simulink model "V126_L8_UMS"  (R2020b)
settings: Solver=VariableStepAuto  StartTime=0.0  StopTime=100  MaxStep=0.04  RelTol=1e-3
undefined symbols (not defined in the file): Ad, Bd, Cd, Dd, F, K, K1, K2, Kg, L, m0, m1, m2, n0, n1, n2, q, T1, T2, T3, Ts, Un
settings Model: Creator=td  LastModifiedBy=Maxim
settings DataIOCC: ReturnWorkspaceOutputs=off
settings DebuggingCC: ArithmeticOperatorsInVariantConditions=warning
settings SFSimCC: CustomCodeUndefinedFunction=UseInterfaceOnly

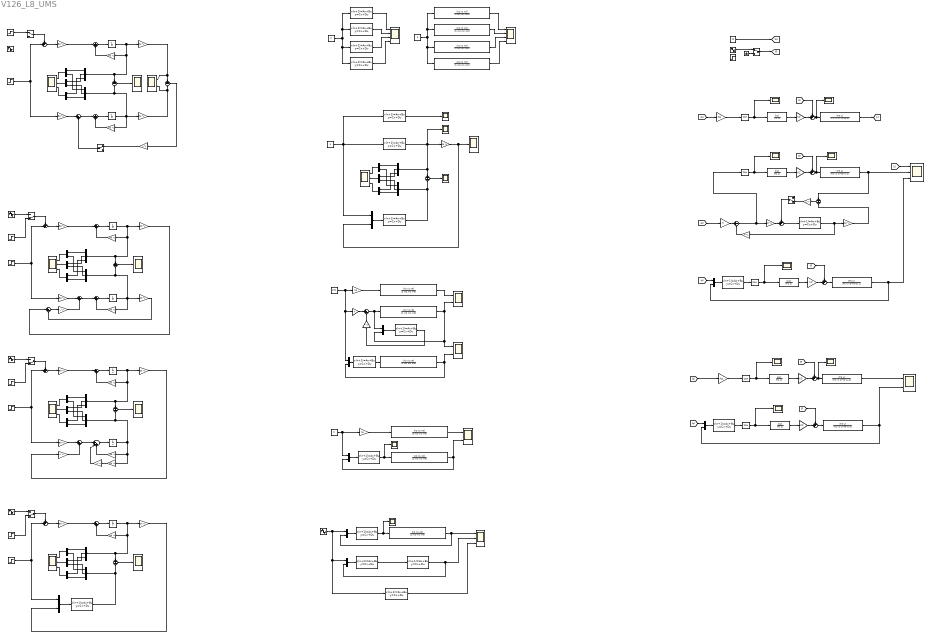
== system V126_L8_UMS ==
  note: Помилка   спостереження
      | вектору     стану
  note: Реальний та спостережений стан об’єкта:
  note: u[n]
  note: ey[n]
  note: x[n+1] = Ad*x[n] + Bd*(u[n]+f[n])
      | y[n] = Cd*x[n]
  note: Збурення f[n]
  note: Модель об'єкта в Просторі Станів
  note: u(t)
  note: V=126; T1=4; T2=6; q=0.3; T3=0.8; K1=0.3; K2=0.2; Un=100;
      |
      | Pn = 6 Bar
      | Rn = 30 rps
      |
      | g = 0.5*Pn = 15 Bar
  note: Вхідні сигнали:
      |
      | g - уставка тиску
      |
      | f - збурення
  note: Об'єкт керування (plant)
  note: Об'єкт керування (plant)
  note: u(t)
  note: xo[n]
  note: Цифрова модель Об'єкта керування (plant) в Просторі Станів
  note: u[n]
  note: Модальний регулятор
  note: u[n]
  note: xo[n+1]
  note: xo[n]
  note: x[n+1]
  note: x[n]
  note: Сигнал
      | керування
  note: y[n]
  note: yo[n]
  note: Спостерігач стану: [Цифровий двійник] + [Корекція помилки спостереження]
  note: ey[n]
  note: ex[n]
  note: x[n]
  note: x[n+1]
  note: xo[n]
  note: xo[n+1]
  note: Модель об'єкта в Просторі Станів
  note: ex[n]
  note: y[n]
  note: Спостерігач стану: [Цифровий двійник] + [Корекція помилки спостереження]
  note: ey[n]
  note: Збурення f[n]
  note: yo[n]
  note: Сигнал
      | керування
  note: x[n+1] = Ad*x[n] + Bd*(u[n]+f[n])
      | y[n] = Cd*x[n]
  note: u[n]
  note: ex[n] = x[n] - xo[n]
      |
      | x[n+1] = A*x[n] + B*u[n]
      | xo[n+1] = A*xo[n] + B*u[n] + L*C*x[n] - L*C*xo[n]
      |
      | x[n+1] - xo[n+1] = A*x[n] + B*u[n] - A*xo[n] - B*u[n] - L*C*x[n] + L*C*xo[n]
      |
      | x[n+1] - xo[n+1] = A*x[n] - L*C*x[n] - A*xo[n] + L*C*xo[n]
      |
      | x[n+1] - xo[n+1] = A*x[n] - L*C*x[n] - (A*xo[n] - L*C*xo[n])
      |
      | x[n+1] - xo[n+1] = (A - L*C)* (x[n] - xo[n])
      |
      | ex[n+1] = (A - L*C)* ex[n]
  note: x[n+1] = A*x[n] + B*u[n]
      | y[n] = C*x[n]
      |
      | xo[n+1] = A*xo[n] + B*u[n]
      | yo[n] = C*xo[n]
  note: xo[n+1] = A*xo[n] + B*u[n] + L (y[n] - yo[n])
      | yo[n] = C*xo[n]
      |
      | xo[n+1] = A*xo[n] + B*u[n] + L (C*x[n] - C*xo[n])
      |
      | xo[n+1] = A*xo[n] + B*u[n] + L*C*x[n] - L*C*xo[n]
      |
      | xo[n+1] = (A - L*C)*xo[n] + B*u[n] + L*C*x[n]
  note: ex[n]
  note: Модель об'єкта в Просторі Станів
  note: xo[n+1]
  note: Спостерігач стану: [Цифровий двійник] + [Корекція помилки спостереження]
  note: y[n]
  note: x[n+1]
  note: x[n]
  note: Сигнал
      | керування
  note: Збурення f[n]
  note: u[n]
  note: xo[n]
  note: x[n+1] = Ad*x[n] + Bd*(u[n]+f[n])
      | y[n] = Cd*x[n]
  note: y[n]
  note: xo[n]
  note: x[n]
  note: xo[n]
  note: Сигнал
      | керування
  note: Спостерігач стану.
  note: y[n]
  note: Збурення f[n]
  note: Модель об'єкта в Просторі Станів
  note: ex[n]
  note: x[n+1] = Ad*x[n] + Bd*(u[n]+f[n])
      | y[n] = Cd*x[n]
  note: y[n]
  note: u[n]
  note: x[n]
  note: x[n]
  note: x[n+1]
  note: xo[n]
  note: ex[n]
  note: x[n]
  note: xo[n]
  note: xo[n]
  note: Спостерігач стану.
  note: x[n]
  note: xo[n]
  note: xo[n+1] = (A - L*C)*xo[n] + B*u[n] + L*y[n]
      | yo[n] = xo[n]
      |
      | ---------------------------------------------------------
      | yr[n] = u[n] = K*g[n] - F*xo[n]
      |
      | xo[n+1] = (A - L*C)*xo[n] + B*(K*g[n] - F*xo[n]) + L*y[n]
      | xo[n+1] = (A - L*C)*xo[n] + B*K*g[n] - B*F*xo[n] + L*y[n]
      |
      | xo[n+1] = (A - L*C-B*F)*xo[n] + B*K*g[n] + L*y[n]
      | yr[n] = -F*xo[n] + K*g[n] + 0*y[n]
  note: u[n]
  note: y[n]
  note: g[n]
  note: u[n]
  note: Об'єкт керування (plant)
  note: u(t)
  note: u[n]
  note: g[n]
  note: y[n]
  note: x[n+1] = Ad*x[n] + Bd*yr[n]
      | y[n] = Cd*x[n]
      |
      | xo[n+1] = (Ad - L*Cd - Bd*F)*xo[n] + Bd*K*u[n] + L*y[n]
      | yr[n] = -F*xo[n] + K*u[n]
      |
      | -------------------------------------------------------------------------------------
      |
      | x[n+1] = Ad*x[n] - Bd*F*xo[n] + Bd*K*u[n]
      | xo[n+1] = L*Cd*x[n] (Ad - L*Cd - Bd*F)*xo[n] + Bd*K*u[n]
      |
      | y[n] = Cd*x[n] + [0,0,0] *xo[n]
  note: u[n]
  note: y[n]
  note: u[n]
  note: y[n]
  note: y[n]
  note: yr[n]
  note: u(t)
  note: Об'єкт керування (plant)
  note: Об'єкт керування (plant)
  note: u(t)
  "    Wpump (s) " : TransferFcn  Numerator=[T3 1]  Denominator=[T2^2 (2*T2*q) 1]
  "    Wpump (s)  " : TransferFcn  Numerator=[T3 1]  Denominator=[T2^2 (2*T2*q) 1]
  "  Wengine (s)  " : TransferFcn  Numerator=[K1]  Denominator=[T1 1]
  "  Wengine (s)   " : TransferFcn  Numerator=[K1]  Denominator=[T1 1]
  "  Wpump (s)" : TransferFcn  Numerator=[T3 1]  Denominator=[T2^2 (2*T2*q) 1]
  "  Wpump (s) " : TransferFcn  Numerator=[T3 1]  Denominator=[T2^2 (2*T2*q) 1]
  "  Wpump (s)   " : TransferFcn  Numerator=[T3 1]  Denominator=[T2^2 (2*T2*q) 1]
  "  y[n]  " : Scope  NumInputPorts=2
  " Plant Model State Space" : DiscreteStateSpace  A=Ad  B=Bd  C=eye(3)  D=[0;0;0]  InitialCondition=[-682.44; 264.94; 115.78]  SampleTime=Ts
  " Plant Model State Space " : DiscreteStateSpace  A=Ad  B=Bd  C=Cd  D=Dd  InitialCondition=[-682.44; 264.94; 115.78]  SampleTime=Ts
  " Plant Model TF " : DiscreteTransferFcn  Numerator=[n2 n1 n0]  Denominator=[1 m2 m1 m0]  InitialStates=[115.78; 264.94; -682.44]  SampleTime=Ts
  " Plant Model TF   " : DiscreteTransferFcn  Numerator=[n2 n1 n0]  Denominator=[1 m2 m1 m0]  InitialStates=[115.78; 264.94; -682.44]  SampleTime=Ts
  " Plant Model TF   1" : DiscreteTransferFcn  Numerator=[n2 n1 n0]  Denominator=[1 m2 m1 m0]  InitialStates=[115.78, 264.94, -682.44]  SampleTime=Ts
  " Plant Model TF   2" : DiscreteTransferFcn  Numerator=[n2 n1 n0]  Denominator=[1 m2 m1 m0]  InitialStates=[0, 0, -1456.6]  SampleTime=Ts
  " Plant Model TF   3" : DiscreteTransferFcn  Numerator=[n2 n1 n0]  Denominator=[1 m2 m1 m0]  InitialStates=[0, 763.7678, 0]  SampleTime=Ts
  " Plant Model TF   4" : DiscreteTransferFcn  Numerator=[n2 n1 n0]  Denominator=[1 m2 m1 m0]  InitialStates=[ 627.2564, 0, 0]  SampleTime=Ts
  " Plant Model1" : DiscreteStateSpace  A=Ad  B=Bd  C=Cd  D=Dd  InitialCondition=[-682.44; 264.94; 115.78]  SampleTime=Ts
  " Plant Model2" : DiscreteStateSpace  A=Ad  B=Bd  C=Cd  D=Dd  InitialCondition=[-1456.6; 0; 0]  SampleTime=Ts
  " Plant Model3" : DiscreteStateSpace  A=Ad  B=Bd  C=Cd  D=Dd  InitialCondition=[0; 763.7678; 0]  SampleTime=Ts
  " Plant Model4" : DiscreteStateSpace  A=Ad  B=Bd  C=Cd  D=Dd  InitialCondition=[0; 0; 627.2564]  SampleTime=Ts
  " R = Observer + ModReg" : DiscreteStateSpace  A=Ad - L*Cd - Bd*F  B=[Bd*K, L]  C=-F  D=[K, 0 ]  SampleTime=Ts
  " System" : DiscreteStateSpace  A=[ Ad, -Bd*F; L*Cd, (Ad - L*Cd - Bd*F)]  B=[Bd*K; Bd*K]  C=[Cd, 0, 0, 0]  D=[0]  InitialCondition=[-682.44; 264.94; 115.78; 0; 0; 0]  SampleTime=Ts
  " u[n] " : Scope
  " y[n]" : Scope
  " y[n]1" : Scope  NumInputPorts=4
  " y[n]2" : Scope  NumInputPorts=2
  " y[n]3" : Scope  NumInputPorts=2
  " y[n]6" : Scope  NumInputPorts=3
  " y[n]7" : Scope
  " y[n]8" : Scope  NumInputPorts=4
  " Порівняльник  " : Scope  NumInputPorts=2
   Порівняльник {1,3,5,8..9,11,13..21} (15 alike) : Scope
   Порівняльник {2,6..7,10,12} (5 alike) : Scope  NumInputPorts=3
  " Порівняльник 4" : Scope  NumInputPorts=2
  -C1 : Step  Time=26  After=-4  SampleTime=0
  -K*Un : Step  Time=26  After=-0.4*Un  SampleTime=0
  Cl/Op Loop Obs : ManualSwitch
  Constant : Constant  Value=0
  Constant1 : Constant  Value=0
  Constant2 : Constant  Value=0
  Constant3 : Constant  Value=12
  Demux{2..11} (10 alike) : Demux  Outputs=3
  Gain{,5,7,9,39} (5 alike) : Gain  Gain=K2
  Gain{1,4,6,8} (4 alike) : Gain  Gain=Kg
  Gain{2,10,12,17,22,24,29,31,37} (9 alike) : Gain  Gain=Cd  Multiplication=Matrix(K*u)
  Gain{11,16,19,23,26,30,33,40} (8 alike) : Gain  Gain=Bd  Multiplication=Matrix(K*u)
  Gain{13,18,25,32,36} (5 alike) : Gain  Gain=L  Multiplication=Matrix(K*u)
  Gain14 : Gain  Gain=F  Multiplication=Matrix(K*u)
  Gain15 : Gain  Gain=K
  Gain{20..21,27..28,34..35,41} (7 alike) : Gain  Gain=Ad  Multiplication=Matrix(K*u)
  Gain3 : Gain  Gain=F  Multiplication=Matrix(K*u)
  Gain38 : Gain  Gain=K
  Ground : Ground
  Manual Switch1 : ManualSwitch
  Manual Switch2 : ManualSwitch
  Manual Switch{3..6} (4 alike) : ManualSwitch  CurrentSetting=0
  Mux{,1..23} (24 alike) : Mux  Inputs=2
  Observer : DiscreteStateSpace  A=Ad-L*Cd  B=[Bd, L]  C=eye(3)  D=[0 0; 0 0; 0 0 ]  SampleTime=Ts
  "Observer " : DiscreteStateSpace  A=Ad-L*Cd  B=[Bd, L]  C=eye(3)  D=[0 0; 0 0; 0 0 ]  SampleTime=Ts
  Observer Cl_Loop : DiscreteStateSpace  A=Ad-L*Cd  B=[Bd, L]  C=eye(3)  D=[0 0; 0 0; 0 0 ]  SampleTime=Ts
  Observer Op_Loop : DiscreteStateSpace  A=Ad  B=Bd  C=eye(3)  D=[0;0;0]  SampleTime=Ts
  Plant Model TF : DiscreteTransferFcn  Numerator=[n2 n1 n0]  Denominator=[1 m2 m1 m0]  InitialStates=[115.78; 264.94; -682.44]  SampleTime=Ts
  "Plant Model TF " : DiscreteTransferFcn  Numerator=[n2 n1 n0]  Denominator=[1 m2 m1 m0]  InitialStates=[115.78; 264.94; -682.44]  SampleTime=Ts
  "Plant Model TF    " : DiscreteTransferFcn  Numerator=[n2 n1 n0]  Denominator=[1 m2 m1 m0]  InitialStates=[115.78; 264.94; -682.44]  SampleTime=Ts
  "Plant Model TF     " : DiscreteTransferFcn  Numerator=[n2 n1 n0]  Denominator=[1 m2 m1 m0]  InitialStates=[115.78; 264.94; -682.44]  SampleTime=Ts
  R = Observer + ModReg : DiscreteStateSpace  A=Ad - L*Cd - Bd*F  B=[Bd*K, L]  C=-F  D=[K, 0 ]  SampleTime=Ts
  "R = Observer + ModReg " : DiscreteStateSpace  A=Ad - L*Cd - Bd*F  B=[Bd*K, L]  C=-F  D=[K, 0 ]  SampleTime=Ts
  "R = Observer + ModReg  " : DiscreteStateSpace  A=Ad - L*Cd - Bd*F  B=[Bd*K, L]  C=-F  D=[K, 0 ]  SampleTime=Ts
  R = Observer + ModReg1 : DiscreteStateSpace  A=Ad - L*Cd - Bd*F  B=[Bd*K, L]  C=-F  D=[K, 0 ]  SampleTime=Ts
  R = Observer + ModReg2 : DiscreteStateSpace  A=Ad - L*Cd - Bd*F  B=[Bd*K, L]  C=-F  D=[K, 0 ]  SampleTime=Ts
  Sine Wave : Sin  Amplitude=2  Frequency=0.4  SampleTime=Ts
  Sine Wave{2..5} (4 alike) : Sin  Amplitude=8  Frequency=0.2  SampleTime=Ts
  Sine Wave6 : Sin  Amplitude=4  Frequency=0.2  SampleTime=0
  Sum : Sum  Inputs=|+-
  Sum{1..2,4..5,7,9..10,21,27,31} (10 alike) : Sum  Inputs=++|
  Sum{11..12,14,16..17,19,22,25,29} (9 alike) : Sum  Inputs=|++
  Sum{3,6,13,15,20,26,30} (7 alike) : Sum  Inputs=+|-
  Sum18 : Sum  Inputs=|+-
  Sum23 : Sum  Inputs=||+-+
  Sum8 : Sum  Inputs=|+-
  Un{,1..2,4} (4 alike) : Step  Time=0  After=Un  SampleTime=0
  Un3 : Step  Time=26  After=-0.4*Un  SampleTime=0
  Un5 : Step  Time=26  After=-0.4*Un  SampleTime=0
  Un6 : Step  Time=26  After=-0.4*Un  SampleTime=0
  Unit Delay{1..6,8} (7 alike) : UnitDelay  SampleTime=Ts  HasFrameUpgradeWarning=on
  "Wengine (s) " : TransferFcn  Numerator=[K1]  Denominator=[T1 1]
  "Wengine (s)  " : TransferFcn  Numerator=[K1]  Denominator=[T1 1]
  "Wengine (s)   " : TransferFcn  Numerator=[K1]  Denominator=[T1 1]
  ZOH : ZeroOrderHold  SampleTime=Ts
  ZOH :) : ZeroOrderHold  SampleTime=Ts
  ZOH :)1 : ZeroOrderHold  SampleTime=Ts
  "ZOH " : ZeroOrderHold  SampleTime=Ts
  ZOH1 : ZeroOrderHold  SampleTime=Ts
  g : Constant  Value=100
  g1 : Constant  Value=0
  x[n+1]=Ad*x[n+1] : DiscreteStateSpace  A="[ 0 1 0 ; 0 0 1 ;  -m0  -m1  -m2 ]"  B=[1 0 0; 0 1 0; 0 0 1]  C=[1 0 0; 0 1 0; 0 0 1]  D=[0 0 0; 0 0 0; 0 0 0]  SampleTime=Ts
  Порівняльник1 : Scope  NumInputPorts=3
  wires:
  Sine Wave6/1 -> Manual Switch1/1
  Gain/1 -> Sum10/2
  Sum10/1 -> " Порівняльник 18"/1, "  Wpump (s)"/1
  Manual Switch1/1 -> [f]
  "  Wpump (s)"/1 -> [y]
  [f] -> Sum10/1
  Constant3/1 -> [g]
  "Wengine (s) "/1 -> Gain/1
  ZOH/1 -> "Wengine (s) "/1, " Порівняльник 3"/1
  Ground/1 -> Manual Switch1/2
  [g] -> Gain1/1
  Gain1/1 -> ZOH/1
  Manual Switch6/1 -> Sum7/1
  "    Wpump (s) "/1 -> Порівняльник1/3, Mux20/2
  Gain9/1 -> Sum5/2
  "Wengine (s)   "/1 -> Gain9/1
  "  Wpump (s)   "/1 -> Порівняльник1/2, Sum6/1
  Gain12/1 -> Sum6/2
  Sum5/1 -> " Порівняльник 17"/1, "  Wpump (s)   "/1
  Gain11/1 -> Sum7/2
  x[n+1]=Ad*x[n+1]/1 -> Gain14/1, Gain12/1
  Sum6/1 -> Gain13/1
  [f] -> Sum5/1
  "ZOH "/1 -> "Wengine (s)   "/1, " Порівняльник 1"/1
  Sum7/1 -> x[n+1]=Ad*x[n+1]/1
  Sum8/1 -> Gain11/1, "ZOH "/1
  Gain14/1 -> Sum8/2
  [g] -> Gain15/1
  Gain15/1 -> Sum8/1
  Unit Delay2/1 -> Gain20/1, Demux2/1, Sum15/1, Gain10/1
  Gain10/1 -> " Порівняльник 4"/1, Sum13/1
  Un/1 -> Sum9/2, Gain16/1
  Unit Delay1/1 -> Demux3/1, Sum15/2, Gain17/1, Gain21/1
  Gain17/1 -> " Порівняльник 4"/2, Sum13/2
  Gain21/1 -> Sum12/2
  Sum11/1 -> Sum12/1
  Sum12/1 -> Unit Delay1/1
  Gain16/1 -> Sum11/1
  -K*Un/1 -> Manual Switch2/1
  Sum9/1 -> Gain19/1
  Manual Switch2/1 -> Sum9/1
  Demux2/1 -> Mux/1
  Demux3/1 -> Mux/2
  Mux/1 -> " Порівняльник 2"/1
  Mux1/1 -> " Порівняльник 2"/2
  Demux3/3 -> Mux2/2
  Mux2/1 -> " Порівняльник 2"/3
  Demux2/3 -> Mux2/1
  Demux2/2 -> Mux1/1
  Demux3/2 -> Mux1/2
  Gain18/1 -> Cl/Op Loop Obs/1
  Cl/Op Loop Obs/1 -> Sum11/2
  Sum13/1 -> Gain18/1
  Sum14/1 -> Unit Delay2/1
  Gain20/1 -> Sum14/2
  Gain19/1 -> Sum14/1
  Sum15/1 -> " Порівняльник 5"/1
  Gain23/1 -> Sum16/1
  Unit Delay4/1 -> Gain27/1, Demux4/1, Sum20/1, Gain22/1
  Gain27/1 -> Sum19/2
  Sum17/1 -> Unit Delay3/1
  Unit Delay3/1 -> Demux5/1, Sum20/2, Gain24/1, Gain28/1
  Gain28/1 -> Sum17/2
  Gain22/1 -> Sum18/1
  Un3/1 -> Manual Switch3/2
  Un2/1 -> Sum21/2, Gain23/1
  Gain26/1 -> Sum19/1
  Demux5/3 -> Mux5/2
  Mux5/1 -> " Порівняльник 6"/3
  Mux4/1 -> " Порівняльник 6"/2
  Sum20/1 -> " Порівняльник 8"/1
  Sum21/1 -> Gain26/1
  Mux3/1 -> " Порівняльник 6"/1
  Demux4/3 -> Mux5/1
  Sine Wave3/1 -> Manual Switch3/1
  Demux5/1 -> Mux3/2
  Demux4/1 -> Mux3/1
  Demux5/2 -> Mux4/2
  Demux4/2 -> Mux4/1
  Sum19/1 -> Unit Delay4/1
  Sum16/1 -> Sum17/1
  Manual Switch3/1 -> Sum21/1
  Gain25/1 -> Sum16/2
  Sum18/1 -> Gain25/1
  Gain24/1 -> Sum18/2
  Mux8/1 -> " Порівняльник 7"/3
  Gain32/1 -> Sum22/2
  Mux7/1 -> " Порівняльник 7"/2
  Gain29/1 -> Gain32/1
  Unit Delay6/1 -> Gain34/1, Demux6/1, Sum26/1, Gain29/1
  Gain34/1 -> Sum25/2
  Demux7/3 -> Mux8/2
  Unit Delay5/1 -> Demux7/1, Sum26/2, Gain37/1, Gain35/1
  Sum26/1 -> " Порівняльник 9"/1
  Gain33/1 -> Sum25/1
  Un4/1 -> Sum27/2, Gain30/1
  Manual Switch4/1 -> Sum27/1
  Sum25/1 -> Unit Delay6/1
  Sum27/1 -> Gain33/1
  Gain30/1 -> Sum22/1
  Demux6/2 -> Mux7/1
  Demux7/2 -> Mux7/2
  Sum23/1 -> Unit Delay5/1
  Demux6/1 -> Mux6/1
  Sine Wave4/1 -> Manual Switch4/1
  Demux6/3 -> Mux8/1
  Demux7/1 -> Mux6/2
  Mux6/1 -> " Порівняльник 7"/1
  Un5/1 -> Manual Switch4/2
  Sum22/1 -> Sum23/1
  Gain35/1 -> Sum23/3
  Gain37/1 -> Gain36/1
  Gain36/1 -> Sum23/2
  Unit Delay8/1 -> Gain41/1, Demux8/1, Sum30/1, Gain31/1
  Demux9/2 -> Mux10/2
  Demux8/2 -> Mux10/1
  Un6/1 -> Manual Switch5/2
  Demux8/1 -> Mux9/1
  Demux8/3 -> Mux11/1
  Manual Switch5/1 -> Sum31/1
  Sum30/1 -> " Порівняльник 11"/1
  Demux9/3 -> Mux11/2
  Demux9/1 -> Mux9/2
  Mux9/1 -> " Порівняльник 10"/1
  Gain31/1 -> Mux12/2
  Un1/1 -> Mux12/1, Sum31/2
  Mux11/1 -> " Порівняльник 10"/3
  Sum29/1 -> Unit Delay8/1
  Gain41/1 -> Sum29/2
  Mux10/1 -> " Порівняльник 10"/2
  Sine Wave2/1 -> Manual Switch5/1
  Sum31/1 -> Gain40/1
  Gain40/1 -> Sum29/1
  Mux12/1 -> Observer/1
  Observer/1 -> Sum30/2, Demux9/1
  Mux13/1 -> " Порівняльник 12"/2
  Mux14/1 -> " Порівняльник 12"/3
  Demux11/1 -> Mux16/2
  Mux16/1 -> " Порівняльник 12"/1
  Demux11/3 -> Mux14/2
  Sum3/1 -> " Порівняльник 13"/1
  Demux10/3 -> Mux14/1
  Demux10/2 -> Mux13/1
  Demux10/1 -> Mux16/1
  " Plant Model State Space"/1 -> " Порівняльник 14"/1, Demux10/1, Sum3/1, Gain2/1
  Demux11/2 -> Mux13/2
  Mux15/1 -> Observer Cl_Loop/1
  Constant/1 -> Observer Op_Loop/1, Mux15/1, " Plant Model State Space"/1
  Observer Cl_Loop/1 -> Sum3/2, Demux11/1
  Gain2/1 -> " y[n]"/1, Mux15/2
  Observer Op_Loop/1 -> " Порівняльник 15"/1
  Constant1/1 -> " Plant Model2"/1, " Plant Model1"/1, " Plant Model4"/1, " Plant Model3"/1
  " Plant Model1"/1 -> " y[n]1"/1
  " Plant Model2"/1 -> " y[n]1"/2
  " Plant Model3"/1 -> " y[n]1"/3
  " Plant Model4"/1 -> " y[n]1"/4
  g/1 -> Mux18/1, Gain38/1, Gain8/1
  Mux17/1 -> "Observer "/1
  Sum/1 -> Mux17/1, " Plant Model TF "/1
  " Plant Model TF "/1 -> " y[n]3"/1, Mux17/2, " y[n]2"/2
  Plant Model TF/1 -> " y[n]2"/1
  Gain3/1 -> Sum/2
  "Observer "/1 -> Gain3/1
  Gain8/1 -> Plant Model TF/1
  Gain38/1 -> Sum/1
  Mux18/1 -> R = Observer + ModReg/1
  R = Observer + ModReg/1 -> "Plant Model TF "/1
  "Plant Model TF "/1 -> " y[n]3"/2, Mux18/2
  "R = Observer + ModReg  "/1 -> " u[n] "/1, "Plant Model TF    "/1
  Mux19/1 -> "R = Observer + ModReg  "/1
  g1/1 -> Gain4/1, Mux19/1
  "Plant Model TF    "/1 -> "  y[n]  "/2, Mux19/2
  " Plant Model TF   "/1 -> "  y[n]  "/1
  R = Observer + ModReg2/1 -> ZOH :)/1
  Gain39/1 -> Sum4/2
  ZOH :)/1 -> " Порівняльник 16"/1, "  Wengine (s)  "/1
  [f] -> Sum4/1
  "  Wengine (s)  "/1 -> Gain39/1
  Sum4/1 -> "    Wpump (s) "/1
  Mux20/1 -> R = Observer + ModReg2/1
  [g] -> Mux20/1
  Gain13/1 -> Manual Switch6/2
  [y] -> Порівняльник1/1
  Gain4/1 -> " Plant Model TF   "/1
  Mux21/1 -> "R = Observer + ModReg "/1
  "R = Observer + ModReg "/1 -> " y[n]7"/1, "Plant Model TF     "/1
  "Plant Model TF     "/1 -> " y[n]6"/1, Mux21/2
  Sine Wave/1 -> " System"/1, Mux22/1, Mux21/1
  " R = Observer + ModReg"/1 -> " Plant Model State Space "/1
  Mux22/1 -> " R = Observer + ModReg"/1
  " Plant Model State Space "/1 -> Mux22/2, " y[n]6"/2
  " System"/1 -> " y[n]6"/3
  " Plant Model TF   1"/1 -> " y[n]8"/1
  " Plant Model TF   2"/1 -> " y[n]8"/2
  " Plant Model TF   3"/1 -> " y[n]8"/3
  " Plant Model TF   4"/1 -> " y[n]8"/4
  Constant2/1 -> " Plant Model TF   3"/1, " Plant Model TF   4"/1, " Plant Model TF   2"/1, " Plant Model TF   1"/1
  "Wengine (s)  "/1 -> Gain5/1
  Sum1/1 -> " Порівняльник 19"/1, "  Wpump (s) "/1
  Gain6/1 -> ZOH1/1
  "  Wpump (s) "/1 -> " Порівняльник  "/1
  Gain5/1 -> Sum1/2
  ZOH1/1 -> "Wengine (s)  "/1, " Порівняльник 20"/1
  [g] -> Gain6/1
  [f] -> Sum1/1
  [g] -> Mux23/1
  Mux23/1 -> R = Observer + ModReg1/1
  "    Wpump (s)  "/1 -> " Порівняльник  "/2, Mux23/2
  Sum2/1 -> "    Wpump (s)  "/1
  "  Wengine (s)   "/1 -> Gain7/1
  ZOH :)1/1 -> " Порівняльник 21"/1, "  Wengine (s)   "/1
  [f] -> Sum2/1
  R = Observer + ModReg1/1 -> ZOH :)1/1
  Gain7/1 -> Sum2/2
